simulink subsystem "Final_Project"  (R2024a)
settings: Solver=VariableStepAuto  StartTime=0.0  StopTime=10.0  RelTol=1e-3
undefined symbols (not defined in the file or in its folder): waypoints
libraries: CarMaker4SL x82
(part 1 of 4)
settings Model: Creator=junho.lee  LastModifiedBy=User

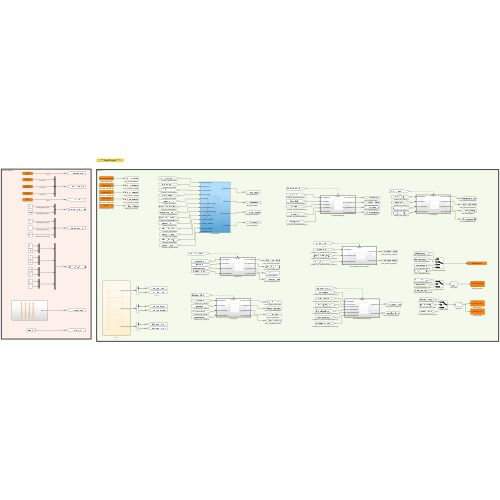
[thumbnail: Simulink's stored preview of the top-level diagram]
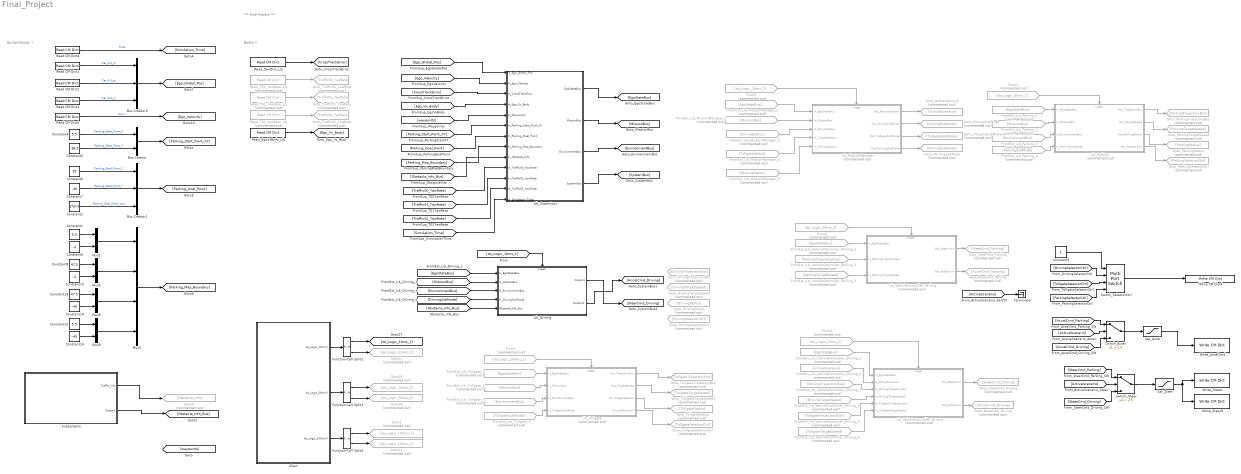
== system Final_Project ==
  note: Do Not Modify !!
  note: *** Final Project ***
  note: Modify !!
  Bus Creator : BusCreator  Inputs=2
  Bus Creator1 : BusCreator  Inputs=3
  Bus Creator3 : BusCreator  Inputs=3
  Chart : Stateflow chart  TreatAsAtomicUnit=on
  Constant1 : Constant  Value=5.5
  Constant10 : Constant  Value=-4
  Constant13 : Constant  Value=47.5
  Constant14 : Constant  Value=-45
  Constant15 : Constant  Value=5.5
  Constant16 : Constant  Value=-45
  Constant2 : Constant  Value=2*pi/3
  Constant3 : Constant
  Constant4 : Constant  Value=5.5
  Constant5 : Constant  Value=-36.5
  Constant6 : Constant  Value=35
  Constant7 : Constant  Value=-30
  Constant8 : Constant  Value=47.5
  Constant9 : Constant  Value=-4
  From1 : From  Commented=on  GotoTag=do_Logic_100ms_1
  From2 : From  Commented=on  GotoTag=do_Logic_50ms_1
  From3 : From  Commented=on  GotoTag=do_Logic_10ms_2
  From4 : From  Commented=on  GotoTag=do_Logic_50ms_2
  From5 : From  Commented=on  GotoTag=do_Logic_10ms_1
  FromExt_Lib_MissionManager_1 : From  Commented=on  GotoTag=EgoStateBus
  FromExt_Lib_MissionManager_2 : From  Commented=on  GotoTag=MissionBus
  FromExt_Lib_MissionManager_3 : From  Commented=on  GotoTag=DrivingStatus
  FromExt_Lib_MissionManager_4 : From  Commented=on  GotoTag=TollgateStatus
  FromExt_Lib_MissionManager_5 : From  Commented=on  GotoTag=ParkingStatus
  FromExt_Lib_Parking_1 : From  Commented=on  GotoTag=EgoStateBus
  FromExt_Lib_Parking_2 : From  Commented=on  GotoTag=MissionBus
  FromExt_Lib_Parking_3 : From  Commented=on  GotoTag=EnvironmentBus
  FromExt_Lib_Parking_4 : From  Commented=on  GotoTag=ParkingSubMode
  FromExt_Lib_Tollgate_1 : From  Commented=on  GotoTag=EgoStateBus
  FromExt_Lib_Tollgate_2 : From  Commented=on  GotoTag=MissionBus
  FromExt_Lib_Tollgate_3 : From  Commented=on  GotoTag=EnvironmentBus
  FromExt_Lib_Tollgate_4 : From  Commented=on  GotoTag=TollgateSubMode
  FromExt_Lib_VehicleController_Driving_1 : From  Commented=on  GotoTag=EgoStateBus
  FromExt_Lib_VehicleController_Driving_2 : From  Commented=on  GotoTag=ActiveScenario
  FromExt_Lib_VehicleController_Driving_3 : From  Commented=on  GotoTag=DrivingTrajectoryBus
  FromExt_Lib_VehicleController_Driving_4 : From  Commented=on  GotoTag=DrivingTargetSpeed
  FromExt_Lib_VehicleController_Driving_5 : From  Commented=on  GotoTag=TollgateTrajectoryBus
  FromExt_Lib_VehicleController_Driving_6 : From  Commented=on  GotoTag=TollgateTargetSpeed
  FromExt_Lib_VehicleController_Parking_1 : From  Commented=on  GotoTag=EgoStateBus
  FromExt_Lib_VehicleController_Parking_2 : From  Commented=on  GotoTag=ParkingTrajectoryBus
  FromExt_Lib_VehicleController_Parking_3 : From  Commented=on  GotoTag=ParkingTargetSpeed
  Function-Call Split1 : FunctionCallSplit  IconShape=distinctive  NumOutputPorts=2  OutputPortLayout=default
  Function-Call Split2 : FunctionCallSplit  IconShape=distinctive  NumOutputPorts=2  OutputPortLayout=default
  Function-Call Split4 : FunctionCallSplit  IconShape=distinctive  NumOutputPorts=2  OutputPortLayout=default
  Goto11 : Goto  Commented=on  GotoTag=do_Logic_100ms_2
  Goto28 : Goto  Commented=on  GotoTag=do_Logic_50ms_1
  Goto3 : Goto  Commented=on  GotoTag=do_Logic_100ms_1
  Goto30 : Goto  Commented=on  GotoTag=do_Logic_50ms_2
  Goto31 : Goto  Commented=on  GotoTag=do_Logic_10ms_2
  Goto9 : Goto  Commented=on  GotoTag=Obstacle_Info
  Goto_AccelCmd_Driving : Goto  Commented=on  GotoTag=AccelCmd_Driving
  Goto_AccelCmd_Parking : Goto  Commented=on  GotoTag=AccelCmd_Parking
  Goto_ActiveScenario : Goto  Commented=on  GotoTag=ActiveScenario
  Goto_DrivingSelectorCtrl : Goto  Commented=on  GotoTag=DrivingSelectorCtrl
  Goto_DrivingStatus : Goto  Commented=on  GotoTag=DrivingStatus
  Goto_DrivingSubMode : Goto  Commented=on  GotoTag=DrivingSubMode
  Goto_DrivingTargetSpeed : Goto  Commented=on  GotoTag=DrivingTargetSpeed
  Goto_DrivingTrajectoryBus : Goto  Commented=on  GotoTag=DrivingTrajectoryBus
  Goto_ParkingSelectorCtrl : Goto  Commented=on  GotoTag=ParkingSelectorCtrl
  Goto_ParkingStatus : Goto  Commented=on  GotoTag=ParkingStatus
  Goto_ParkingSubMode : Goto  Commented=on  GotoTag=ParkingSubMode
  Goto_ParkingTargetSpeed : Goto  Commented=on  GotoTag=ParkingTargetSpeed
  Goto_ParkingTrajectoryBus : Goto  Commented=on  GotoTag=ParkingTrajectoryBus
  Goto_SteerCmd_Driving : Goto  Commented=on  GotoTag=SteerCmd_Driving
  Goto_SteerCmd_Parking : Goto  Commented=on  GotoTag=SteerCmd_Parking
  Goto_TollgateSelectorCtrl : Goto  Commented=on  GotoTag=TollgateSelectorCtrl
  Goto_TollgateStatus : Goto  Commented=on  GotoTag=TollgateStatus
  Goto_TollgateSubMode : Goto  Commented=on  GotoTag=TollgateSubMode
  Goto_TollgateTargetSpeed : Goto  Commented=on  GotoTag=TollgateTargetSpeed
  Goto_TollgateTrajectoryBus : Goto  Commented=on  GotoTag=TollgateTrajectoryBus
  Goto_Traffic00_YawRate : Goto  Commented=on  GotoTag=Traffic00_YawRate
  Goto_Traffic01_YawRate : Goto  Commented=on  GotoTag=Traffic01_YawRate
  Goto_Traffic02_YawRate : Goto  Commented=on  GotoTag=Traffic02_YawRate
  Lib_Driving : Subsystem
  Lib_MissionManager : Subsystem  Commented=on
  Lib_Parking : Subsystem  Commented=on
  Lib_Supervisor : Subsystem
  Lib_Tollgate : Subsystem  Commented=on
  Lib_VehicleController_Driving : Subsystem  Commented=on
  Lib_VehicleController_Parking : Subsystem  Commented=on
  Mux{2,5,8..9} (4 alike) : Mux  Inputs=2
  Mux4 : Mux
  Read CM Dict1 : CarMaker4SL/Read CM Dict  xname=Car.Fr1.tx  xsync=off  xstime=Inherited
  Read CM Dict2 : CarMaker4SL/Read CM Dict  xname=Car.Fr1.ty  xsync=off  xstime=Inherited
  Read CM Dict3 : CarMaker4SL/Read CM Dict  xname=Car.Fr1.rz  xsync=off  xstime=Inherited
  Read CM Dict4 : CarMaker4SL/Read CM Dict  xname=Time  xsync=off  xstime=Inherited
  Read CM Dict5 : CarMaker4SL/Read CM Dict  xname=Car.v  xsync=off  xstime=Inherited
  Read_DevDist_Lib : CarMaker4SL/Read CM Dict  xname=Car.Road.Path.DevDist  xsync=off  xstime=Inherited
  Read_EgoVxBody_Lib : CarMaker4SL/Read CM Dict  xname=Car.vx  xsync=off  xstime=Inherited
  Read_T00_YawRate_Lib : CarMaker4SL/Read CM Dict  Commented=on  xname=Traffic.T00.rzv  xsync=off  xstime=Inherited
  Read_T01_YawRate_Lib : CarMaker4SL/Read CM Dict  Commented=on  xname=Traffic.T01.rzv  xsync=off  xstime=Inherited
  Read_T02_YawRate_Lib : CarMaker4SL/Read CM Dict  Commented=on  xname=Traffic.T02.rzv  xsync=off  xstime=Inherited
  Sat_Accel : Saturate  UpperLimit=3.0  LowerLimit=-5.0
  Sat_Steer : Saturate  UpperLimit=pi/6  LowerLimit=-pi/6
  Subsystem1 : Subsystem
  Switch_Accel : Switch  Criteria=u2 > Threshold  Threshold=2.5
  Switch_SelectorCtrl : MultiPortSwitch  DataPortOrder=Specify indices  DataPortIndices={1, 2, 3}  OutDataTypeStr=double
  Switch_Steer : Switch  Criteria=u2 > Threshold  Threshold=2.5
  Terminator : Terminator
  Write CM Dict4 : CarMaker4SL/Write CM Dict  xname=DM.SelectorCtrl  xsync=off
  Write_AccelCmd : CarMaker4SL/Write CM Dict  xname=AccelCtrl.DesiredAx  xsync=off
  Write_SteerL : CarMaker4SL/Write CM Dict  xname=Car.CFL.rz_ext  xsync=off
  Write_SteerR : CarMaker4SL/Write CM Dict  xname=Car.CFR.rz_ext  xsync=off
  wires:
  Constant13/1 -> Mux8/1
  Subsystem1/1(Traffic_Info) -> Goto9/1
  Read CM Dict1/1 -> Bus Creator3/1  "Car_Fr1_tx"
  Read CM Dict3/1 -> Bus Creator3/3  "Car_Fr1_rz"
  Constant4/1 -> Bus Creator/1  "Parking_Start_Point_X"
  Chart/2(do_Logic_50ms()) -> Function-Call Split1/1
  Function-Call Split2/1 -> [do_Logic_10ms_1]
  Function-Call Split1/2 -> Goto30/1
  Read CM Dict4/1 -> [Simulation_Time]  "Time"
  Constant9/1 -> Mux2/2
  Bus Creator1/1 -> [Parking_Goal_Point]
  Mux8/1 -> Mux4/3
  Constant6/1 -> Bus Creator1/1  "Parking_Goal_Point_X"
  Constant1/1 -> Mux2/1
  Constant16/1 -> Mux9/2
  Read CM Dict2/1 -> Bus Creator3/2  "Car_Fr1_ty"
  Function-Call Split1/1 -> Goto28/1
  Constant5/1 -> Bus Creator/2  "Parking_Start_Point_Y"
  Chart/1(do_Logic_10ms()) -> Function-Call Split2/1
  Constant7/1 -> Bus Creator1/2  "Parking_Goal_Point_Y"
  Read CM Dict5/1 -> [Ego_Velocity]  "Car.v"
  Constant15/1 -> Mux9/1
  Constant10/1 -> Mux5/2
  Bus Creator3/1 -> [Ego_Global_Pos]
  Constant14/1 -> Mux8/2
  Function-Call Split2/2 -> Goto31/1
  Bus Creator/1 -> [Parking_Start_Point_XY]
  Mux9/1 -> Mux4/4
  Mux2/1 -> Mux4/1
  Mux4/1 -> [Parking_Map_Boundary]
  Constant8/1 -> Mux5/1
  Constant2/1 -> Bus Creator1/3  "Parking_Goal_Point_Yaw"
  Mux5/1 -> Mux4/2
  Chart/3(do_Logic_100ms()) -> Function-Call Split4/1
  Function-Call Split4/1 -> Goto3/1
  Function-Call Split4/2 -> Goto11/1
  Sat_Steer/1 -> Write_SteerR/1, Write_SteerL/1
  Read_DevDist_Lib/1 -> [CrossTrackError]
  Read_T00_YawRate_Lib/1 -> Goto_Traffic00_YawRate/1
  Read_T01_YawRate_Lib/1 -> Goto_Traffic01_YawRate/1
  Read_T02_YawRate_Lib/1 -> Goto_Traffic02_YawRate/1
  Read_EgoVxBody_Lib/1 -> [Ego_Vx_Body]
  [Ego_Global_Pos] -> Lib_Supervisor/1(In_Ego_Global_Pos)
  [Ego_Velocity] -> Lib_Supervisor/2(In_Ego_Velocity)
  [CrossTrackError] -> Lib_Supervisor/3(In_CrossTrackError)
  [Ego_Vx_Body] -> Lib_Supervisor/4(In_Ego_Vx_Body)
  [waypoints] -> Lib_Supervisor/5(In_Waypoints)
  [Parking_Start_Point_XY] -> Lib_Supervisor/6(In_Parking_Start_Point_XY)
  [Parking_Goal_Point] -> Lib_Supervisor/7(In_Parking_Goal_Point)
  [Parking_Map_Boundary] -> Lib_Supervisor/8(In_Parking_Map_Boundary)
  [Traffic00_YawRate] -> Lib_Supervisor/10(In_Traffic00_YawRate)
  [Traffic01_YawRate] -> Lib_Supervisor/11(In_Traffic01_YawRate)
  [Traffic02_YawRate] -> Lib_Supervisor/12(In_Traffic02_YawRate)
  [Simulation_Time] -> Lib_Supervisor/13(In_Simulation_Time)
  Lib_Supervisor/1(EgoStateBus) -> [EgoStateBus]
  Lib_Supervisor/2(MissionBus) -> [MissionBus]
  Lib_Supervisor/3(EnvironmentBus) -> [EnvironmentBus]
  Lib_Supervisor/4(SystemBus) -> [SystemBus]
  Lib_MissionManager/1(Out_ActiveScenario) -> Goto_ActiveScenario/1
  Lib_MissionManager/2(Out_DrivingSubMode) -> Goto_DrivingSubMode/1
  Lib_MissionManager/3(Out_TollgateSubMode) -> Goto_TollgateSubMode/1
  Lib_MissionManager/4(Out_ParkingSubMode) -> Goto_ParkingSubMode/1
  Lib_Tollgate/1(Out_TrajectoryBus) -> Goto_TollgateTrajectoryBus/1
  Lib_Tollgate/2(Out_TargetSpeed) -> Goto_TollgateTargetSpeed/1
  Lib_Tollgate/3(Out_TollgateStatus) -> Goto_TollgateStatus/1
  Lib_Parking/1(Out_TrajectoryBus) -> Goto_ParkingTrajectoryBus/1
  Lib_Parking/2(Out_TargetSpeed) -> Goto_ParkingTargetSpeed/1
  Lib_Parking/3(Out_ParkingStatus) -> Goto_ParkingStatus/1
  Lib_VehicleController_Driving/1(Out_SteerCmd) -> Goto_SteerCmd_Driving/1
  Lib_VehicleController_Driving/2(Out_AccelCmd) -> Goto_AccelCmd_Driving/1
  Lib_VehicleController_Parking/1(Out_SteerCmd) -> Goto_SteerCmd_Parking/1
  Lib_VehicleController_Parking/2(Out_AccelCmd) -> Goto_AccelCmd_Parking/1
  FromExt_Lib_MissionManager_1/1 -> Lib_MissionManager/1(In_EgoStateBus)
  FromExt_Lib_MissionManager_2/1 -> Lib_MissionManager/2(In_MissionBus)
  FromExt_Lib_MissionManager_3/1 -> Lib_MissionManager/3(In_DrivingStatus)
  FromExt_Lib_MissionManager_4/1 -> Lib_MissionManager/4(In_TollgateStatus)
  FromExt_Lib_MissionManager_5/1 -> Lib_MissionManager/5(In_ParkingStatus)
  [EgoStateBus] -> Lib_Driving/1(In_EgoStateBus)
  [MissionBus] -> Lib_Driving/2(In_MissionBus)
  [EnvironmentBus] -> Lib_Driving/3(In_EnvironmentBus)
  [DrivingSubMode] -> Lib_Driving/4(In_DrivingSubMode)
  FromExt_Lib_Tollgate_1/1 -> Lib_Tollgate/1(In_EgoStateBus)
  FromExt_Lib_Tollgate_2/1 -> Lib_Tollgate/2(In_MissionBus)
  FromExt_Lib_Tollgate_3/1 -> Lib_Tollgate/3(In_EnvironmentBus)
  FromExt_Lib_Tollgate_4/1 -> Lib_Tollgate/4(In_TollgateSubMode)
  FromExt_Lib_Parking_1/1 -> Lib_Parking/1(In_EgoStateBus)
  FromExt_Lib_Parking_2/1 -> Lib_Parking/2(In_MissionBus)
  FromExt_Lib_Parking_3/1 -> Lib_Parking/3(In_EnvironmentBus)
  FromExt_Lib_Parking_4/1 -> Lib_Parking/4(In_ParkingSubMode)
  FromExt_Lib_VehicleController_Driving_1/1 -> Lib_VehicleController_Driving/1(In_EgoStateBus)
  FromExt_Lib_VehicleController_Driving_2/1 -> Lib_VehicleController_Driving/2(In_ActiveScenario)
  FromExt_Lib_VehicleController_Driving_3/1 -> Lib_VehicleController_Driving/3(In_DrivingTrajectoryBus)
  FromExt_Lib_VehicleController_Driving_4/1 -> Lib_VehicleController_Driving/4(In_DrivingTargetSpeed)
  FromExt_Lib_VehicleController_Driving_5/1 -> Lib_VehicleController_Driving/5(In_TollgateTrajectoryBus)
  FromExt_Lib_VehicleController_Driving_6/1 -> Lib_VehicleController_Driving/6(In_TollgateTargetSpeed)
  FromExt_Lib_VehicleController_Parking_1/1 -> Lib_VehicleController_Parking/1(In_EgoStateBus)
  FromExt_Lib_VehicleController_Parking_2/1 -> Lib_VehicleController_Parking/2(In_ParkingTrajectoryBus)
  FromExt_Lib_VehicleController_Parking_3/1 -> Lib_VehicleController_Parking/3(In_ParkingTargetSpeed)
  From5/1 -> Lib_MissionManager/Trigger
  From3/1 -> Lib_VehicleController_Driving/Trigger
  From4/1 -> Lib_VehicleController_Parking/Trigger
  [do_Logic_10ms_1] -> Lib_Driving/Trigger
  From1/1 -> Lib_Tollgate/Trigger
  From2/1 -> Lib_Parking/Trigger
  [SteerCmd_Parking] -> Switch_Steer/1
  [ActiveScenario] -> Switch_Steer/2
  [SteerCmd_Driving] -> Switch_Steer/3
  Switch_Steer/1 -> Sat_Steer/1
  [AccelCmd_Parking] -> Switch_Accel/1
  [ActiveScenario] -> Switch_Accel/2
  [AccelCmd_Driving] -> Switch_Accel/3
  Switch_Accel/1 -> Sat_Accel/1
  Lib_Tollgate/4(Out_SelectorCtrl) -> Goto_TollgateSelectorCtrl/1
  Lib_Parking/4(Out_SelectorCtrl) -> Goto_ParkingSelectorCtrl/1
  [DrivingSelectorCtrl] -> Switch_SelectorCtrl/2
  [TollgateSelectorCtrl] -> Switch_SelectorCtrl/3
  [ParkingSelectorCtrl] -> Switch_SelectorCtrl/4
  Switch_SelectorCtrl/1 -> Write CM Dict4/1
  Constant3/1 -> Switch_SelectorCtrl/1
  [ActiveScenario] -> Terminator/1
  Sat_Accel/1 -> Write_AccelCmd/1
  Subsystem1/2(Outport) -> [Obstacle_Info_Bus]
  [Obstacle_Info_Bus] -> Lib_Supervisor/9(In_Obstacle_Info)
  Lib_Driving/1(Outport) -> [SteerCmd_Driving]
  Lib_Driving/2(Outport1) -> [AccelCmd_Driving]
  [Obstacle_Info_Bus] -> Lib_Driving/5(Obstacle_Info_Bus)

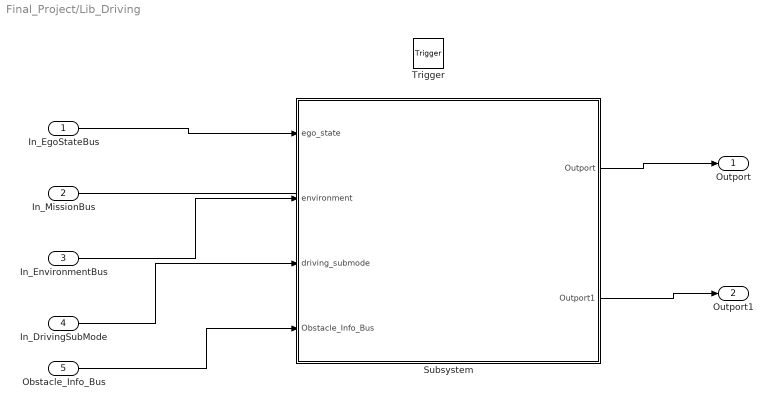
== system Final_Project/Lib_Driving ==
  In_EgoStateBus : Inport
  In_MissionBus : Inport  Port=2
  In_EnvironmentBus : Inport  Port=3
  In_DrivingSubMode : Inport  Port=4
  Obstacle_Info_Bus : Inport  Port=5
  Trigger : TriggerPort  TriggerType=function-call  VariantControl=(inherit)
  Subsystem : Subsystem
  Outport : Outport
  Outport1 : Outport  Port=2
  wires:
  Obstacle_Info_Bus/1 -> Subsystem/4(Obstacle_Info_Bus)
  Subsystem/2(Outport1) -> Outport1/1
  Subsystem/1(Outport) -> Outport/1
  In_DrivingSubMode/1 -> Subsystem/3(driving_submode)
  In_EgoStateBus/1 -> Subsystem/1(ego_state)
  In_EnvironmentBus/1 -> Subsystem/2(environment)
  In_MissionBus/1 -> ?

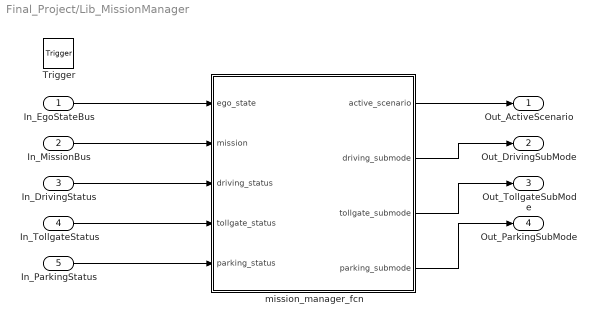
== system Final_Project/Lib_MissionManager ==
  In_EgoStateBus : Inport
  In_MissionBus : Inport  Port=2
  In_DrivingStatus : Inport  Port=3
  In_TollgateStatus : Inport  Port=4
  In_ParkingStatus : Inport  Port=5
  Trigger : TriggerPort  TriggerType=function-call  VariantControl=(inherit)
  mission_manager_fcn : MATLAB Function  TreatAsAtomicUnit=on
  Out_ActiveScenario : Outport
  Out_DrivingSubMode : Outport  Port=2
  Out_TollgateSubMode : Outport  Port=3
  Out_ParkingSubMode : Outport  Port=4
  wires:
  In_EgoStateBus/1 -> mission_manager_fcn/1(ego_state)
  In_MissionBus/1 -> mission_manager_fcn/2(mission)
  In_DrivingStatus/1 -> mission_manager_fcn/3(driving_status)
  In_TollgateStatus/1 -> mission_manager_fcn/4(tollgate_status)
  In_ParkingStatus/1 -> mission_manager_fcn/5(parking_status)
  mission_manager_fcn/1(active_scenario) -> Out_ActiveScenario/1
  mission_manager_fcn/2(driving_submode) -> Out_DrivingSubMode/1
  mission_manager_fcn/3(tollgate_submode) -> Out_TollgateSubMode/1
  mission_manager_fcn/4(parking_submode) -> Out_ParkingSubMode/1

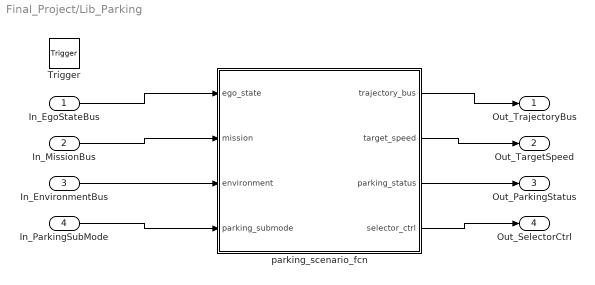
== system Final_Project/Lib_Parking ==
  In_EgoStateBus : Inport
  In_MissionBus : Inport  Port=2
  In_EnvironmentBus : Inport  Port=3
  In_ParkingSubMode : Inport  Port=4
  Trigger : TriggerPort  TriggerType=function-call  VariantControl=(inherit)
  parking_scenario_fcn : MATLAB Function  TreatAsAtomicUnit=on
  Out_TrajectoryBus : Outport
  Out_TargetSpeed : Outport  Port=2
  Out_ParkingStatus : Outport  Port=3
  Out_SelectorCtrl : Outport  Port=4
  wires:
  In_EgoStateBus/1 -> parking_scenario_fcn/1(ego_state)
  In_MissionBus/1 -> parking_scenario_fcn/2(mission)
  In_EnvironmentBus/1 -> parking_scenario_fcn/3(environment)
  In_ParkingSubMode/1 -> parking_scenario_fcn/4(parking_submode)
  parking_scenario_fcn/1(trajectory_bus) -> Out_TrajectoryBus/1
  parking_scenario_fcn/2(target_speed) -> Out_TargetSpeed/1
  parking_scenario_fcn/3(parking_status) -> Out_ParkingStatus/1
  parking_scenario_fcn/4(selector_ctrl) -> Out_SelectorCtrl/1

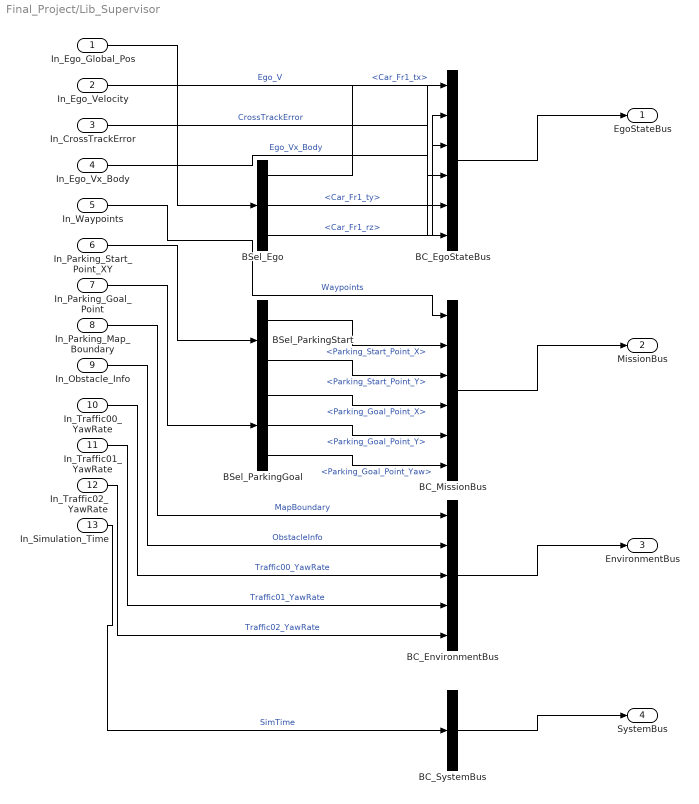
== system Final_Project/Lib_Supervisor ==
  In_Ego_Global_Pos : Inport
  In_Ego_Velocity : Inport  Port=2
  In_CrossTrackError : Inport  Port=3
  In_Ego_Vx_Body : Inport  Port=4
  In_Waypoints : Inport  Port=5
  In_Parking_Start_Point_XY : Inport  Port=6
  In_Parking_Goal_Point : Inport  Port=7
  In_Parking_Map_Boundary : Inport  Port=8
  In_Obstacle_Info : Inport  Port=9
  In_Traffic00_YawRate : Inport  Port=10
  In_Traffic01_YawRate : Inport  Port=11
  In_Traffic02_YawRate : Inport  Port=12
  In_Simulation_Time : Inport  Port=13
  BC_EgoStateBus : BusCreator  Inputs=6
  BC_EnvironmentBus : BusCreator  Inputs=5
  BC_MissionBus : BusCreator  Inputs=6
  BC_SystemBus : BusCreator  Inputs=1
  BSel_Ego : BusSelector  OutputSignals=Car_Fr1_tx,Car_Fr1_ty,Car_Fr1_rz
  BSel_ParkingGoal : BusSelector  OutputSignals=Parking_Goal_Point_X,Parking_Goal_Point_Y,Parking_Goal_Point_Yaw
  BSel_ParkingStart : BusSelector  OutputSignals=Parking_Start_Point_X,Parking_Start_Point_Y
  EgoStateBus : Outport
  MissionBus : Outport  Port=2
  EnvironmentBus : Outport  Port=3
  SystemBus : Outport  Port=4
  wires:
  In_Ego_Global_Pos/1 -> BSel_Ego/1
  In_Parking_Start_Point_XY/1 -> BSel_ParkingStart/1
  In_Parking_Goal_Point/1 -> BSel_ParkingGoal/1
  BSel_Ego/1 -> BC_EgoStateBus/1  "<Car_Fr1_tx>"
  BSel_Ego/2 -> BC_EgoStateBus/2  "<Car_Fr1_ty>"
  BSel_Ego/3 -> BC_EgoStateBus/3  "<Car_Fr1_rz>"
  In_Ego_Velocity/1 -> BC_EgoStateBus/4  "Ego_V"
  In_CrossTrackError/1 -> BC_EgoStateBus/5  "CrossTrackError"
  In_Ego_Vx_Body/1 -> BC_EgoStateBus/6  "Ego_Vx_Body"
  In_Waypoints/1 -> BC_MissionBus/1  "Waypoints"
  BSel_ParkingStart/1 -> BC_MissionBus/2  "<Parking_Start_Point_X>"
  BSel_ParkingStart/2 -> BC_MissionBus/3  "<Parking_Start_Point_Y>"
  BSel_ParkingGoal/1 -> BC_MissionBus/4  "<Parking_Goal_Point_X>"
  BSel_ParkingGoal/2 -> BC_MissionBus/5  "<Parking_Goal_Point_Y>"
  BSel_ParkingGoal/3 -> BC_MissionBus/6  "<Parking_Goal_Point_Yaw>"
  In_Parking_Map_Boundary/1 -> BC_EnvironmentBus/1  "MapBoundary"
  In_Obstacle_Info/1 -> BC_EnvironmentBus/2  "ObstacleInfo"
  In_Traffic00_YawRate/1 -> BC_EnvironmentBus/3  "Traffic00_YawRate"
  In_Traffic01_YawRate/1 -> BC_EnvironmentBus/4  "Traffic01_YawRate"
  In_Traffic02_YawRate/1 -> BC_EnvironmentBus/5  "Traffic02_YawRate"
  In_Simulation_Time/1 -> BC_SystemBus/1  "SimTime"
  BC_EgoStateBus/1 -> EgoStateBus/1
  BC_MissionBus/1 -> MissionBus/1
  BC_EnvironmentBus/1 -> EnvironmentBus/1
  BC_SystemBus/1 -> SystemBus/1

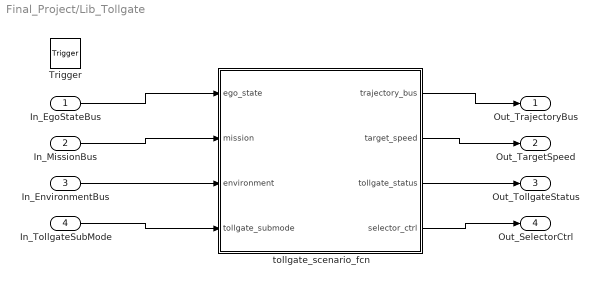
== system Final_Project/Lib_Tollgate ==
  In_EgoStateBus : Inport
  In_MissionBus : Inport  Port=2
  In_EnvironmentBus : Inport  Port=3
  In_TollgateSubMode : Inport  Port=4
  Trigger : TriggerPort  TriggerType=function-call  VariantControl=(inherit)
  tollgate_scenario_fcn : MATLAB Function  TreatAsAtomicUnit=on
  Out_TrajectoryBus : Outport
  Out_TargetSpeed : Outport  Port=2
  Out_TollgateStatus : Outport  Port=3
  Out_SelectorCtrl : Outport  Port=4
  wires:
  In_EgoStateBus/1 -> tollgate_scenario_fcn/1(ego_state)
  In_MissionBus/1 -> tollgate_scenario_fcn/2(mission)
  In_EnvironmentBus/1 -> tollgate_scenario_fcn/3(environment)
  In_TollgateSubMode/1 -> tollgate_scenario_fcn/4(tollgate_submode)
  tollgate_scenario_fcn/1(trajectory_bus) -> Out_TrajectoryBus/1
  tollgate_scenario_fcn/2(target_speed) -> Out_TargetSpeed/1
  tollgate_scenario_fcn/3(tollgate_status) -> Out_TollgateStatus/1
  tollgate_scenario_fcn/4(selector_ctrl) -> Out_SelectorCtrl/1

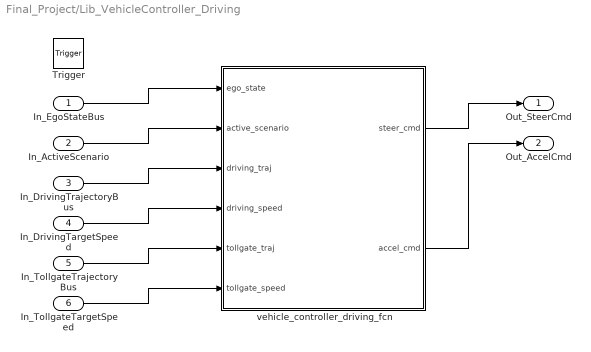
== system Final_Project/Lib_VehicleController_Driving ==
  In_EgoStateBus : Inport
  In_ActiveScenario : Inport  Port=2
  In_DrivingTrajectoryBus : Inport  Port=3
  In_DrivingTargetSpeed : Inport  Port=4
  In_TollgateTrajectoryBus : Inport  Port=5
  In_TollgateTargetSpeed : Inport  Port=6
  Trigger : TriggerPort  TriggerType=function-call  VariantControl=(inherit)
  vehicle_controller_driving_fcn : MATLAB Function  TreatAsAtomicUnit=on
  Out_SteerCmd : Outport
  Out_AccelCmd : Outport  Port=2
  wires:
  In_EgoStateBus/1 -> vehicle_controller_driving_fcn/1(ego_state)
  In_ActiveScenario/1 -> vehicle_controller_driving_fcn/2(active_scenario)
  In_DrivingTrajectoryBus/1 -> vehicle_controller_driving_fcn/3(driving_traj)
  In_DrivingTargetSpeed/1 -> vehicle_controller_driving_fcn/4(driving_speed)
  In_TollgateTrajectoryBus/1 -> vehicle_controller_driving_fcn/5(tollgate_traj)
  In_TollgateTargetSpeed/1 -> vehicle_controller_driving_fcn/6(tollgate_speed)
  vehicle_controller_driving_fcn/1(steer_cmd) -> Out_SteerCmd/1
  vehicle_controller_driving_fcn/2(accel_cmd) -> Out_AccelCmd/1

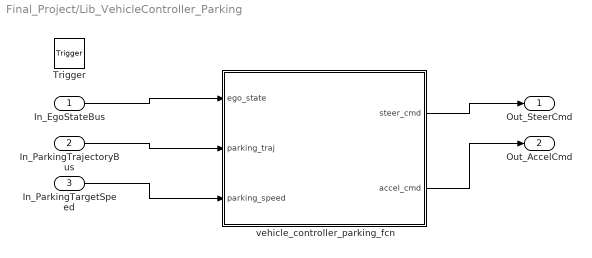
== system Final_Project/Lib_VehicleController_Parking ==
  In_EgoStateBus : Inport
  In_ParkingTrajectoryBus : Inport  Port=2
  In_ParkingTargetSpeed : Inport  Port=3
  Trigger : TriggerPort  TriggerType=function-call  VariantControl=(inherit)
  vehicle_controller_parking_fcn : MATLAB Function  TreatAsAtomicUnit=on
  Out_SteerCmd : Outport
  Out_AccelCmd : Outport  Port=2
  wires:
  In_EgoStateBus/1 -> vehicle_controller_parking_fcn/1(ego_state)
  In_ParkingTrajectoryBus/1 -> vehicle_controller_parking_fcn/2(parking_traj)
  In_ParkingTargetSpeed/1 -> vehicle_controller_parking_fcn/3(parking_speed)
  vehicle_controller_parking_fcn/1(steer_cmd) -> Out_SteerCmd/1
  vehicle_controller_parking_fcn/2(accel_cmd) -> Out_AccelCmd/1
